simulink model "dstr_algorithm"  (R2019b)
settings: Solver=VariableStepAuto  StartTime=0.0  StopTime=200  RelTol=1e-3
values from neighbouring files (symbols this model uses):
  Am1 = 1 - 1.3205 + 0.4966    (= 0.1761)    [dstr_demo.m]
  am1 = -1.3205    [discrete1.m]    (also in discrete2.m; dstr_demo.m; istr.m)
  am2 = 0.4966    [discrete1.m]    (also in discrete2.m; dstr_demo.m; istr.m)
  lambda = 0.95    [discrete1.m]    (also in dstr_demo.m = 0.98; istr.m = 0.1)
  P_0 = eye(4,4) * 100    [dstr_demo.m]
  theta_init = [.4,.3,.1,-.4]'    [dstr_demo.m]
  Ts = 1    [ProportionalController.m]    (also in RLS_demo_init.m = 1e-05; dstr_demo.m = 0.5)
libraries: dspmtrx3 x1
settings Model: Creator=jaber  LastModifiedBy=jaber

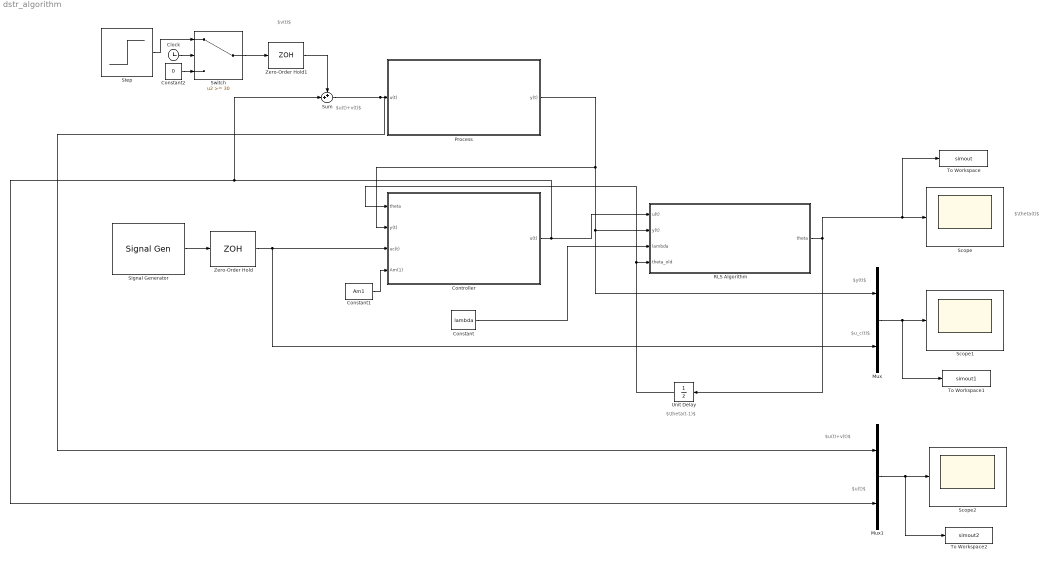
== system dstr_algorithm ==
  note: $u(t)+v(t)$
  note: $\theta(t-1)$
  note: $\theta(t)$
  note: $v(t)$
  note: $y(t)$
  note: $u_c(t)$
  note: $u(t)$
  note: $u(t)+v(t)$
  Clock : Clock
  Constant : Constant  Value=lambda
  Constant1 : Constant  Value=Am1
  Constant2 : Constant  Value=0
  Controller : Subsystem
  Mux : Mux  Inputs=2
  Mux1 : Mux  Inputs=2
  "Process " : Subsystem
  "RLS Algorithm " : Subsystem
  Scope : Scope
  Scope1 : Scope
  Scope2 : Scope
  Signal Generator : SignalGenerator  WaveForm=square  Amplitude=-1  Frequency=1/40
  Step : Step  SampleTime=Ts  ZeroCross=off
  Sum : Sum  Inputs=++|
  Switch : Switch  Threshold=30
  To Workspace : ToWorkspace  VariableName=simout  SaveFormat=Timeseries  SampleTime=-1
  To Workspace1 : ToWorkspace  VariableName=simout1  SaveFormat=Timeseries  SampleTime=-1
  To Workspace2 : ToWorkspace  VariableName=simout2  SaveFormat=Timeseries  SampleTime=-1
  Unit Delay : UnitDelay  InitialCondition=theta_init  SampleTime=-1  HasFrameUpgradeWarning=on
  Zero-Order Hold : ZeroOrderHold  SampleTime=Ts
  Zero-Order Hold1 : ZeroOrderHold  SampleTime=Ts
  wires:
  Controller/1(u(t)) -> Sum/2, Mux1/2, "RLS Algorithm "/1(u(t))
  Constant/1 -> "RLS Algorithm "/3(lambda)
  "RLS Algorithm "/1(theta) -> Unit Delay/1, Scope/1, To Workspace/1
  Constant1/1 -> Controller/4(Am(1))
  Switch/1 -> Zero-Order Hold1/1
  Mux/1 -> To Workspace1/1, Scope1/1
  Unit Delay/1 -> "RLS Algorithm "/4(theta_old), Controller/1(theta)
  "Process "/1(y(t)) -> Controller/2(y(t)), Mux/1, "RLS Algorithm "/2(y(t))
  Signal Generator/1 -> Zero-Order Hold/1
  Zero-Order Hold/1 -> Mux/2, Controller/3(uc(t))
  Sum/1 -> Mux1/1, "Process "/1(u(t))
  Clock/1 -> Switch/2
  Step/1 -> Switch/1
  Constant2/1 -> Switch/3
  Zero-Order Hold1/1 -> Sum/1
  Mux1/1 -> To Workspace2/1, Scope2/1

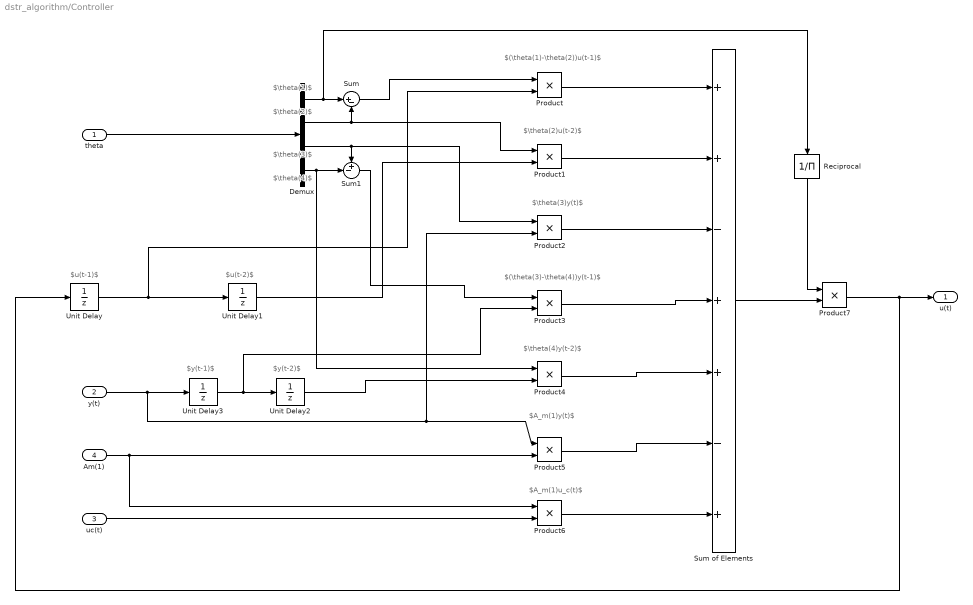
== system dstr_algorithm/Controller ==
  note: $u(t-1)$
  note: $\theta(2)u(t-2)$
  note: $(\theta(1)-\theta(2))u(t-1)$
  note: $\theta(1)$
  note: $\theta(2)$
  note: $\theta(3)$
  note: $\theta(4)$
  note: $u(t-2)$
  note: $\theta(3)y(t)$
  note: $y(t-1)$
  note: $y(t-2)$
  note: $(\theta(3)-\theta(4))y(t-1)$
  note: $\theta(4)y(t-2)$
  note: $A_m(1)y(t)$
  note: $A_m(1)u_c(t)$
  theta : Inport
  y(t) : Inport  Port=2
  uc(t) : Inport  Port=3
  Am(1) : Inport  Port=4
  Demux : Demux
  Product{,1..7} (8 alike) : Product
  Reciprocal : Product  Inputs=/
  Sum : Sum  Inputs=|+-
  Sum of Elements : Sum  Inputs=++-++-+
  Sum1 : Sum  Inputs=+-|
  Unit Delay{,1..3} (4 alike) : UnitDelay  SampleTime=-1  HasFrameUpgradeWarning=on
  u(t) : Outport
  wires:
  theta/1 -> Demux/1
  Demux/2 -> Product1/1, Sum/2
  Sum/1 -> Product/1
  Unit Delay/1 -> Product/2, Unit Delay1/1
  Unit Delay1/1 -> Product1/2
  Demux/4 -> Product4/1, Sum1/2
  Demux/3 -> Product2/1, Sum1/1
  y(t)/1 -> Product5/1, Product2/2, Unit Delay3/1
  Unit Delay3/1 -> Product3/2, Unit Delay2/1
  Sum1/1 -> Product3/1
  Unit Delay2/1 -> Product4/2
  Am(1)/1 -> Product5/2, Product6/1
  uc(t)/1 -> Product6/2
  Product/1 -> Sum of Elements/1
  Product1/1 -> Sum of Elements/2
  Product2/1 -> Sum of Elements/3
  Product3/1 -> Sum of Elements/4
  Product4/1 -> Sum of Elements/5
  Product5/1 -> Sum of Elements/6
  Product6/1 -> Sum of Elements/7
  Product7/1 -> Unit Delay/1, u(t)/1
  Reciprocal/1 -> Product7/1
  Sum of Elements/1 -> Product7/2
  Demux/1 -> Reciprocal/1, Sum/1

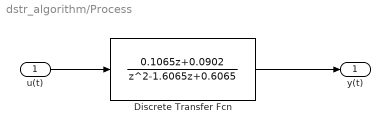
== system dstr_algorithm/Process  ==
  u(t) : Inport
  Discrete Transfer Fcn : DiscreteTransferFcn  Numerator=[0.1065 0.0902]  Denominator=[1 -1.6065 0.6065]
  y(t) : Outport
  wires:
  Discrete Transfer Fcn/1 -> y(t)/1
  u(t)/1 -> Discrete Transfer Fcn/1

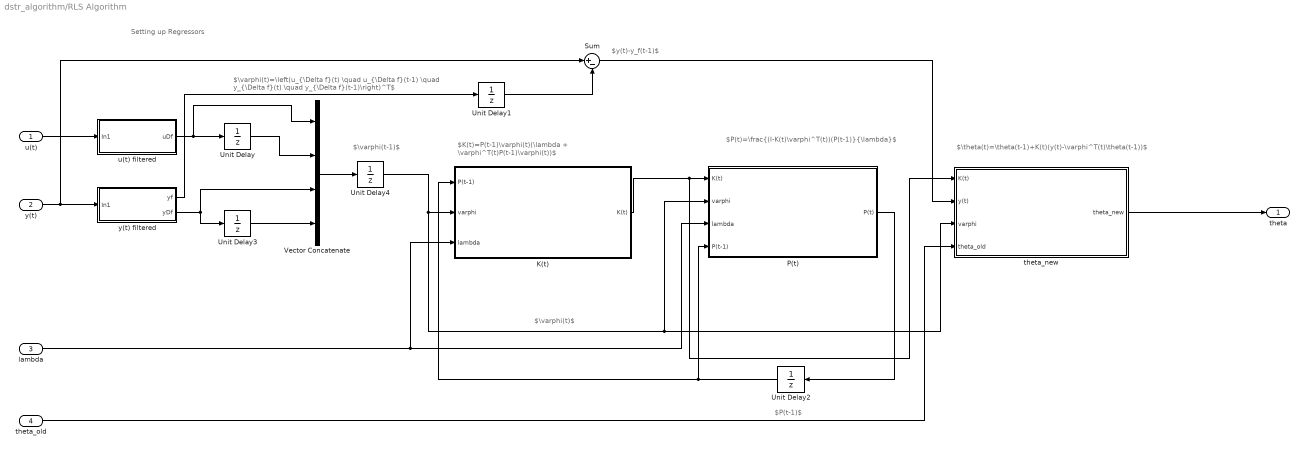
== system dstr_algorithm/RLS Algorithm  ==
  note: $\varphi(t-1)$
  note: $P(t-1)$
  note: $\varphi(t)$
  note: Setting up Regressors
  note: $K(t)=P(t-1)\varphi(t)(\lambda + \varphi^T(t)P(t-1)\varphi(t))$
  note: $\varphi(t)=\left(u_{\Delta f}(t) \quad u_{\Delta f}(t-1) \quad y_{\Delta f}(t) \quad y_{\Delta f}(t-1)\right)^T$
  note: $P(t)=\frac{(I-K(t)\varphi^T(t))(P(t-1)}{\lambda}$
  note: $y(t)-y_f(t-1)$
  note: $\theta(t)=\theta(t-1)+K(t)(y(t)-\varphi^T(t)\theta(t-1))$
  u(t) : Inport
  y(t) : Inport  Port=2
  lambda : Inport  Port=3
  theta_old : Inport  Port=4
  K(t) : Subsystem
  P(t) : Subsystem
  Sum : Sum  Inputs=|+-
  Unit Delay{,1,3..4} (4 alike) : UnitDelay  SampleTime=-1  HasFrameUpgradeWarning=on
  Unit Delay2 : UnitDelay  InitialCondition=P_0  SampleTime=-1  HasFrameUpgradeWarning=on
  Vector Concatenate : Concatenate  NumInputs=4
  theta_new : Subsystem
  u(t) filtered : Subsystem
  y(t) filtered : Subsystem
  theta : Outport
  wires:
  u(t)/1 -> u(t) filtered/1(In1)
  y(t)/1 -> Sum/1, y(t) filtered/1(In1)
  u(t) filtered/1(uDf) -> Vector Concatenate/1, Unit Delay/1
  Unit Delay/1 -> Vector Concatenate/2
  theta_new/1(theta_new) -> theta/1
  Vector Concatenate/1 -> Unit Delay4/1
  P(t)/1(P(t)) -> Unit Delay2/1
  Unit Delay2/1 -> P(t)/4(P(t-1)), K(t)/1(P(t-1))
  lambda/1 -> K(t)/3(lambda), P(t)/3(lambda)
  K(t)/1(K(t)) -> P(t)/1(K(t)), theta_new/1(K(t))
  theta_old/1 -> theta_new/4(theta_old)
  Sum/1 -> theta_new/2(y(t))
  Unit Delay3/1 -> Vector Concatenate/4
  y(t) filtered/2(yDf) -> Vector Concatenate/3, Unit Delay3/1
  y(t) filtered/1(yf) -> Unit Delay1/1
  Unit Delay1/1 -> Sum/2
  Unit Delay4/1 -> P(t)/2(varphi), theta_new/3(varphi), K(t)/2(varphi)

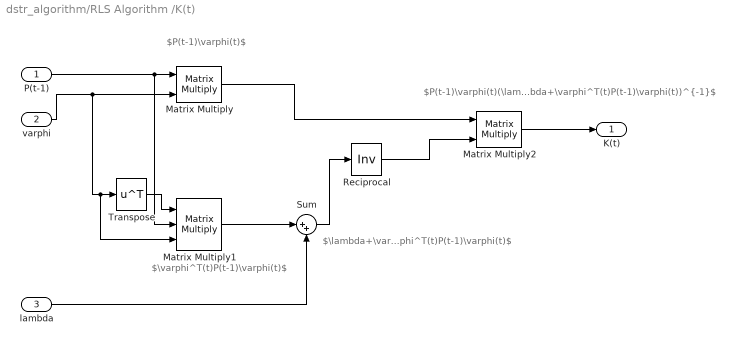
== system dstr_algorithm/RLS Algorithm /K(t) ==
  note: $\lambda+\varphi^T(t)P(t-1)\varphi(t)$
  note: $\varphi^T(t)P(t-1)\varphi(t)$
  note: $P(t-1)\varphi(t)$
  note: $P(t-1)\varphi(t)(\lambda+\varphi^T(t)P(t-1)\varphi(t))^{-1}$
  P(t-1) : Inport
  varphi : Inport  Port=2
  lambda : Inport  Port=3
  Matrix Multiply : Product  Multiplication=Matrix(*)
  Matrix Multiply1 : Product  Inputs=3  Multiplication=Matrix(*)
  Matrix Multiply2 : Product  Multiplication=Matrix(*)
  Reciprocal : Product  Inputs=/  Multiplication=Matrix(*)  SaturateOnIntegerOverflow=on  RndMeth=Zero
  Sum : Sum  Inputs=|++
  Transpose : Math  Operator=transpose  SignedPower=off  SaturateOnIntegerOverflow=on
  K(t) : Outport
  wires:
  P(t-1)/1 -> Matrix Multiply1/2, Matrix Multiply/1
  varphi/1 -> Matrix Multiply/2, Matrix Multiply1/3, Transpose/1
  Transpose/1 -> Matrix Multiply1/1
  lambda/1 -> Sum/2
  Matrix Multiply1/1 -> Sum/1
  Matrix Multiply/1 -> Matrix Multiply2/1
  Matrix Multiply2/1 -> K(t)/1
  Sum/1 -> Reciprocal/1
  Reciprocal/1 -> Matrix Multiply2/2

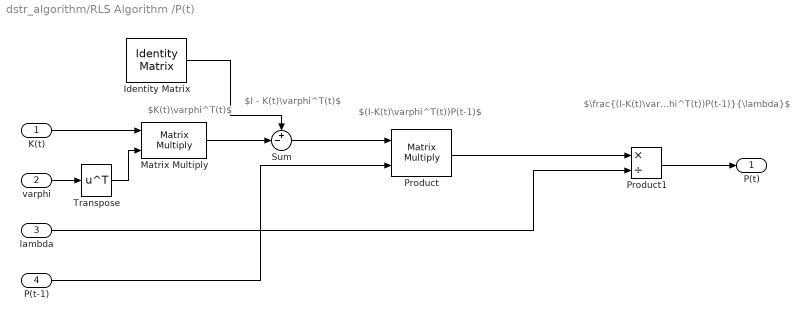
== system dstr_algorithm/RLS Algorithm /P(t) ==
  note: $(I-K(t)\varphi^T(t))P(t-1)$
  note: $I - K(t)\varphi^T(t)$
  note: $\frac{(I-K(t)\varphi^T(t))P(t-1)}{\lambda}$
  note: $K(t)\varphi^T(t)$
  K(t) : Inport
  varphi : Inport  Port=2
  lambda : Inport  Port=3
  P(t-1) : Inport  Port=4
  Identity Matrix : dspmtrx3/Identity Matrix  Inherit=off  N=4  Ts=1  dataType=double  isSigned=on  wordLen=16  udDataType=sfix(16)  fracBitsMode=Best precision  numFracBits=15  OutDataTypeStr=double  LastOutDataTypeStr=double
      settings: SourceProductName=DSP System Toolbox
  Matrix Multiply : Product  Multiplication=Matrix(*)
  Product : Product  Multiplication=Matrix(*)
  Product1 : Product  Inputs=*/
  Sum : Sum  Inputs=+-|
  Transpose : Math  Operator=transpose  SignedPower=off  SaturateOnIntegerOverflow=on
  P(t) : Outport
  wires:
  K(t)/1 -> Matrix Multiply/1
  varphi/1 -> Transpose/1
  Transpose/1 -> Matrix Multiply/2
  lambda/1 -> Product1/2
  Product/1 -> Product1/1
  Product1/1 -> P(t)/1
  P(t-1)/1 -> Product/2
  Matrix Multiply/1 -> Sum/2
  Sum/1 -> Product/1
  Identity Matrix/1 -> Sum/1

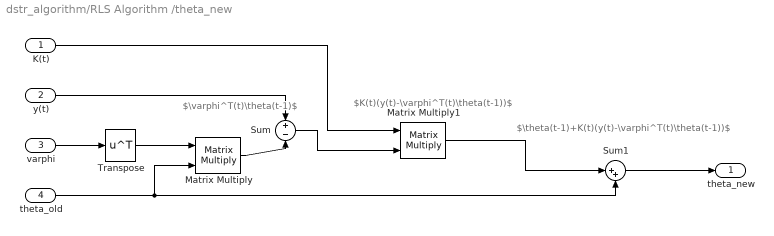
== system dstr_algorithm/RLS Algorithm /theta_new ==
  note: $\varphi^T(t)\theta(t-1)$
  note: $K(t)(y(t)-\varphi^T(t)\theta(t-1))$
  note: $\theta(t-1)+K(t)(y(t)-\varphi^T(t)\theta(t-1))$
  K(t) : Inport
  y(t) : Inport  Port=2
  varphi : Inport  Port=3
  theta_old : Inport  Port=4
  Matrix Multiply : Product  Multiplication=Matrix(*)
  Matrix Multiply1 : Product  Multiplication=Matrix(*)
  Sum : Sum  Inputs=+|-
  Sum1 : Sum  Inputs=|++
  Transpose : Math  Operator=transpose  SignedPower=off  SaturateOnIntegerOverflow=on
  theta_new : Outport
  wires:
  varphi/1 -> Transpose/1
  theta_old/1 -> Sum1/2, Matrix Multiply/2
  Matrix Multiply/1 -> Sum/2
  K(t)/1 -> Matrix Multiply1/1
  Matrix Multiply1/1 -> Sum1/1
  Sum1/1 -> theta_new/1
  Transpose/1 -> Matrix Multiply/1
  y(t)/1 -> Sum/1
  Sum/1 -> Matrix Multiply1/2

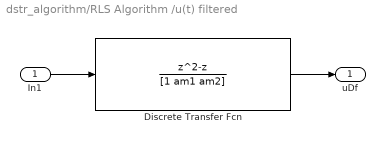
== system dstr_algorithm/RLS Algorithm /u(t) filtered ==
  In1 : Inport
  Discrete Transfer Fcn : DiscreteTransferFcn  Numerator=[1 -1 0]  Denominator=[1 am1 am2]
  uDf : Outport
  wires:
  Discrete Transfer Fcn/1 -> uDf/1
  In1/1 -> Discrete Transfer Fcn/1

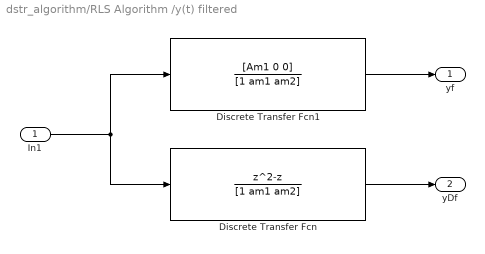
== system dstr_algorithm/RLS Algorithm /y(t) filtered ==
  In1 : Inport
  Discrete Transfer Fcn : DiscreteTransferFcn  Numerator=[1 -1 0]  Denominator=[1 am1 am2]
  Discrete Transfer Fcn1 : DiscreteTransferFcn  Numerator=[Am1 0 0]  Denominator=[1 am1 am2]
  yf : Outport
  yDf : Outport  Port=2
  wires:
  In1/1 -> Discrete Transfer Fcn1/1, Discrete Transfer Fcn/1
  Discrete Transfer Fcn1/1 -> yf/1
  Discrete Transfer Fcn/1 -> yDf/1
